simulink model "Conexion_Inalambrica_2020B"  (R2020b)
settings: Solver=ode1  StartTime=0.0  StopTime=inf  FixedStep=0.009  MaxStep=0.01  RelTol=1e-3
undefined symbols (not defined in the file): LF
libraries: instrumentlib x3, slrealtimeutilitieslib x1
settings Model: PacingRate=0.100000  Creator=ricar  LastModifiedBy=ricar

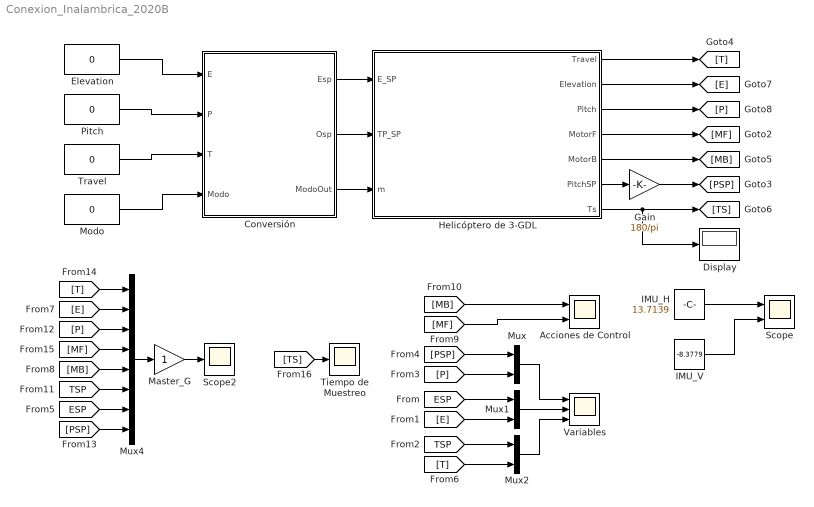
== system Conexion_Inalambrica_2020B ==
  Acciones de Control : Scope  NumInputPorts=2
  Conversión : Subsystem
  Display : Display
  Elevation : Constant  Value=0
  Gain : Gain  Gain=180/pi
  Helicóptero de 3-GDL : Subsystem
      mask Display: image('$imagefile'); % Use "Edit Image" on toolstrip to change.
  IMU_H : Constant  Value=13.7139
  IMU_V : Constant  Value=-8.3779
  Master_G : Gain
  Modo : Constant  Value=0
  Mux : Mux  Inputs=2
  Mux1 : Mux  Inputs=2
  Mux2 : Mux  Inputs=2
  Mux4 : Mux  Inputs=8
  Pitch : Constant  Value=0
  Scope : Scope  NumInputPorts=2
  Scope2 : Scope
  Tiempo de Muestreo : Scope
  Travel : Constant  Value=0
  Variables : Scope  NumInputPorts=3
  wires:
  Mux/1 -> Variables/1
  Mux1/1 -> Variables/2
  Mux2/1 -> Variables/3
  Gain/1 -> [PSP]
  [P] -> Mux/2
  [E] -> Mux1/2
  [T] -> Mux2/2
  [MF] -> Acciones de Control/2
  [MB] -> Acciones de Control/1
  [ESP] -> Mux1/1
  [TSP] -> Mux2/1
  [PSP] -> Mux/1
  [T] -> Mux4/1
  [E] -> Mux4/2
  [P] -> Mux4/3
  [MF] -> Mux4/4
  [MB] -> Mux4/5
  [TSP] -> Mux4/6
  [ESP] -> Mux4/7
  [PSP] -> Mux4/8
  Mux4/1 -> Master_G/1
  Master_G/1 -> Scope2/1
  Modo/1 -> Conversión/4(Modo)
  Helicóptero de 3-GDL/7(Ts) -> [TS], Display/1
  Helicóptero de 3-GDL/4(MotorF) -> [MF]
  Helicóptero de 3-GDL/5(MotorB) -> [MB]
  Helicóptero de 3-GDL/6(PitchSP) -> Gain/1
  Elevation/1 -> Conversión/1(E)
  Pitch/1 -> Conversión/2(P)
  Travel/1 -> Conversión/3(T)
  Conversión/1(Esp) -> Helicóptero de 3-GDL/1(E_SP)
  Conversión/2(Osp) -> Helicóptero de 3-GDL/2(TP_SP)
  Conversión/3(ModoOut) -> Helicóptero de 3-GDL/3(m)
  [TS] -> Tiempo de Muestreo/1
  IMU_H/1 -> Scope/1
  IMU_V/1 -> Scope/2
  Helicóptero de 3-GDL/1(Travel) -> [T]
  Helicóptero de 3-GDL/2(Elevation) -> [E]
  Helicóptero de 3-GDL/3(Pitch) -> [P]

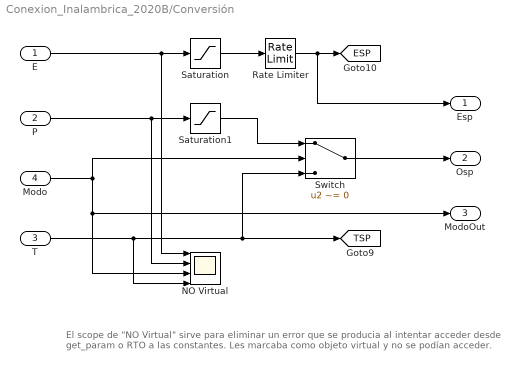
== system Conexion_Inalambrica_2020B/Conversión ==
  note: El scope de "NO Virtual" sirve para eliminar un error que se producia al intentar acceder desde get_param o RTO a las constantes. Les marcaba como objeto virtual y no se podían acceder.
  E : Inport
  P : Inport  Port=2
  T : Inport  Port=3
  Modo : Inport  Port=4
  NO Virtual : Scope  NumInputPorts=4
  Rate Limiter : RateLimiter  RisingSlewLimit=8  FallingSlewLimit=-8  SampleTimeMode=inherited
  Saturation : Saturate  UpperLimit=30  LowerLimit=-28.35
  Saturation1 : Saturate  UpperLimit=20  LowerLimit=-20
  Switch : Switch  Criteria=u2 ~= 0
  Esp : Outport
  Osp : Outport  Port=2
  ModoOut : Outport  Port=3
  tag scope: ESP=global, TSP=global
  wires:
  Saturation/1 -> Rate Limiter/1
  P/1 -> NO Virtual/2, Saturation1/1
  T/1 -> NO Virtual/4, [TSP], Switch/3
  Rate Limiter/1 -> Esp/1, [ESP]
  Modo/1 -> Switch/2, ModoOut/1, NO Virtual/3
  E/1 -> NO Virtual/1, Saturation/1
  Saturation1/1 -> Switch/1
  Switch/1 -> Osp/1

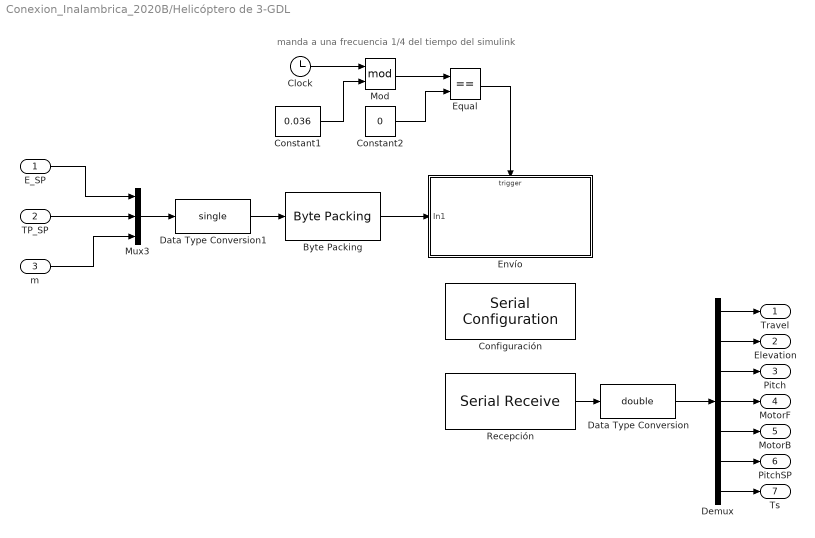
== system Conexion_Inalambrica_2020B/Helicóptero de 3-GDL ==
  note: manda a una frecuencia 1/4 del tiempo del simulink
  E_SP : Inport
  TP_SP : Inport  Port=2
  m : Inport  Port=3
  Byte Packing : slrealtimeutilitieslib/Byte Packing  MaskPackedDataType=uint8  MaskUnpackedDataTypes={'single'}  MaskAlignment=1
  Clock : Clock
  Configuración : instrumentlib/Serial Configuration  Priority=-200000  ObjConstructor=serial('<Select a port...>');  ComPortMenu=<Please select a port...>  ComPort=<Please select a port...>  BaudRate=115200  DataBits=8  Parity=none  StopBits=1  ByteOrder=LittleEndian  FlowControl=none  Timeout=10
  Constant1 : Constant  Value=0.036
  Constant2 : Constant  Value=0
  Data Type Conversion : DataTypeConversion  OutDataTypeStr=double
  Data Type Conversion1 : DataTypeConversion  OutDataTypeStr=single
  Demux : Demux  Outputs=7
  Envío : Subsystem  TreatAsAtomicUnit=on
  Equal : RelationalOperator  Operator===  OutDataTypeStr=boolean  RndMeth=Simplest
  Mod : Math  Operator=mod  SaturateOnIntegerOverflow=on
  Mux3 : Mux  Inputs=3
  Recepción : instrumentlib/Serial Receive  Priority=1  ObjConstructor=serial('<Select a port...>');  ComPortMenu=<Please select a port...>  ComPort=<Please select a port...>  DataType=single  DataSize=[1 7]  EnableBlockingMode=on  ActionDataUnavailable=Output last received value  CustomValue=0  SampleTime=-1
  Travel : Outport
  Elevation : Outport  Port=2
  Pitch : Outport  Port=3
  MotorF : Outport  Port=4
  MotorB : Outport  Port=5
  PitchSP : Outport  Port=6
  Ts : Outport  Port=7
  wires:
  Constant1/1 -> Mod/2
  Equal/1 -> Envío/Trigger
  Data Type Conversion/1 -> Demux/1
  Byte Packing/1 -> Envío/1(In1)
  Data Type Conversion1/1 -> Byte Packing/1
  Clock/1 -> Mod/1
  Constant2/1 -> Equal/2
  Mod/1 -> Equal/1
  Mux3/1 -> Data Type Conversion1/1
  Recepción/1 -> Data Type Conversion/1
  Demux/6 -> PitchSP/1
  TP_SP/1 -> Mux3/2
  Demux/1 -> Travel/1
  Demux/2 -> Elevation/1
  m/1 -> Mux3/3
  Demux/7 -> Ts/1
  E_SP/1 -> Mux3/1
  Demux/3 -> Pitch/1
  Demux/4 -> MotorF/1
  Demux/5 -> MotorB/1

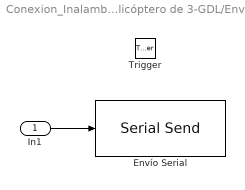
== system Conexion_Inalambrica_2020B/Helicóptero de 3-GDL/Envío ==
  In1 : Inport
  Trigger : TriggerPort  VariantControl=(inherit)
  Envío Serial : instrumentlib/Serial Send  Priority=1  ObjConstructor=serial('<Select a port...>');  ComPortMenu=<Please select a port...>  ComPort=<Please select a port...>  Terminator=LF ('\n')  EnableBlockingMode=off
  wires:
  In1/1 -> Envío Serial/1
